simulink model "SWC_HALIN_type"  (R2021b)
settings: Solver=FixedStepDiscrete  StartTime=0.0  StopTime=10.0  FixedStep=0.005  RelTol=1e-3
values from neighbouring files (symbols this model uses):
  FALSE = boolean( 0 )    [vcu_local_hdr.m]    (also in vcu_local_hdrTA2.m)
  TRUE = boolean( 1 )    [vcu_local_hdr.m]    (also in vcu_local_hdrTA2.m)
undefined symbols (not defined in the file or in its folder): R_WDGCDD_CSOP_Call_Watchdog, R_WDGCDD_CSOP_Call_WDG_AppStart
libraries: halin x1, simulink x1
settings Model: DataDictionary=APPTypes.sldd  Creator=FVT23010  LastModifiedBy=FVT22063
settings DataIOCC: SaveFormat=StructureWithTime
settings OptimizationCC: DefaultParameterBehavior=Inlined  EnhancedBackFolding=on  PassReuseOutputArgsAs=Individual arguments  ZeroExternalMemoryAtStartup=off  ZeroInternalMemoryAtStartup=off  OptimizeBlockOrder=speed  DifferentSizesBufferReuse=on  OptimizationCustomize=off  EfficientTunableParamExpr=on
settings DebuggingCC: ParameterTunabilityLossMsg=error
settings HardwareCC: ProdBitPerPointer=32  ProdBitPerSizeT=32  ProdBitPerPtrDiffT=32  ProdLargestAtomicInteger=Long  ProdLargestAtomicFloat=Double  ProdWordSize=32  ProdLongLongMode=on  ProdHWDeviceType=ARM Compatible->ARM Cortex-M
settings ModelReferenceCC: ModelReferenceNumInstancesAllowed=Single
settings SFSimCC: MATLABDynamicMemAlloc=off
settings RTWCC: Description=AUTOSAR  SystemTargetFile=autosar.tlc  GenCodeOnly=on  TemplateMakefile=ert_default_tmf  PortableWordSizes=on
settings CodeAppCC: ForceParamTrailComments=on  IgnoreCustomStorageClasses=off  OperatorAnnotations=on  SimulinkDataObjDesc=on  SFDataObjDesc=on  InsertBlockDesc=on
settings STFCustomTargetCC: TargetLangStandard=C99 (ISO)  MultiwordLength=256  ParMdlRefBuildCompliant=on  CompOptLevelCompliant=on  IncludeMdlTerminateFcn=off  CombineOutputUpdateFcns=on  SuppressErrorStatus=on  ERTCustomFileBanners=on  SupportNonFinite=off  SupportComplex=off  SupportContinuousTime=off  SupportNonInlinedSFcns=off  RemoveResetFunc=on  MATLABClassNameForMDSCustomization=Simulink.SoftwareTarget.ERTCustomization  AutosarCompliant=on  GRTInterface=off  UseToolchainInfoCompliant=on  LookupTableObjectStructAxisOrder=2,1,3,4,...  LUTObjectStructOrderEvenSpacing=Size,Table,Breakpoints  SystemTargetFile=autosar.tlc
settings ERTTargetCC: TargetLangStandard=C99 (ISO)  ConcurrentExecutionCompliant=off  IncludeMdlTerminateFcn=off  SuppressErrorStatus=on  SupportNonFinite=off  SupportComplex=off  ModelStepFunctionPrototypeControlCompliant=off  CPPClassGenCompliant=off  AutosarCompliant=on  LookupTableObjectStructAxisOrder=2,1,3,4,...  LUTObjectStructOrderEvenSpacing=Size,Table,Breakpoints  GenerateASAP2=on  InlinedParameterPlacement=NonHierarchical  ERTCustomFileTemplate=example_file_process.tlc  ConvertIfToSwitch=off  SuppressUnreachableDefaultCases=off  BooleanTrueId=true_MatlabRTW  BooleanFalseId=false_MatlabRTW

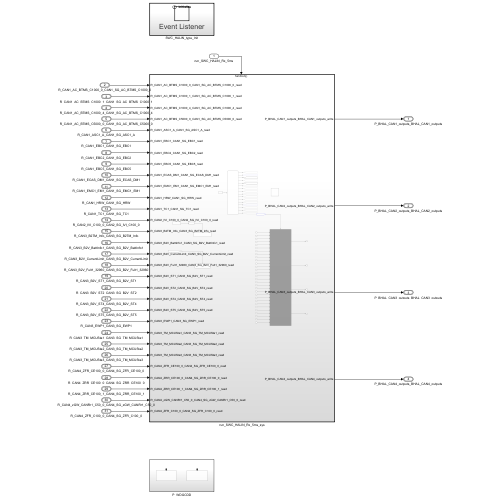
[thumbnail: Simulink's stored preview of the top-level diagram]
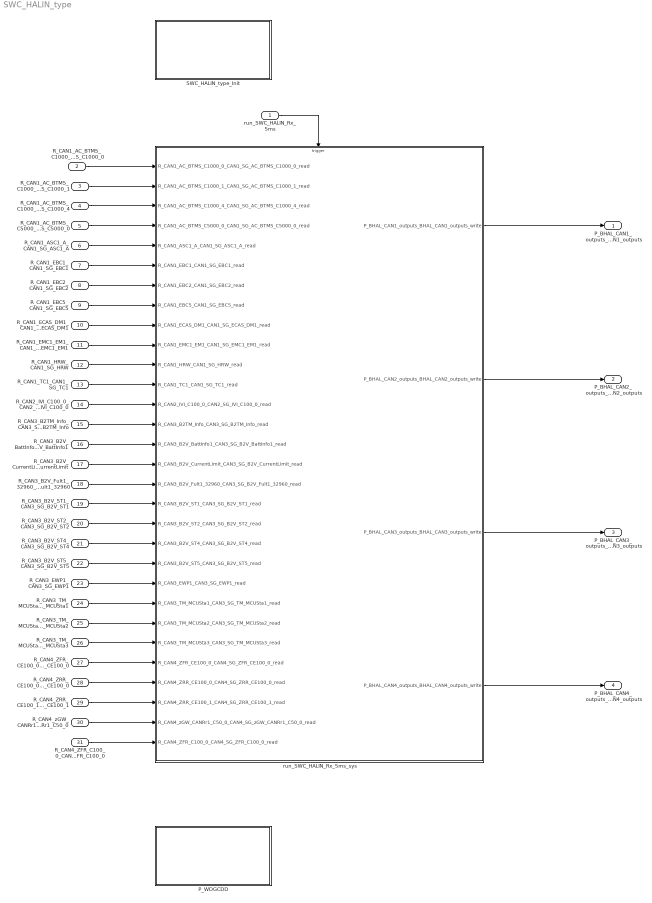
== system SWC_HALIN_type ==
  run_SWC_HALIN_Rx_5ms : Inport  SampleTime=0.005  OutputFunctionCall=on
  R_CAN1_AC_BTMS_C1000_0_CAN1_SG_AC_BTMS_C1000_0 : Inport  Port=2  OutDataTypeStr=Bus: DT_CAN1_SG_AC_BTMS_C1000_0  PortDimensions=1  BusOutputAsStruct=on
  R_CAN1_AC_BTMS_C1000_1_CAN1_SG_AC_BTMS_C1000_1 : Inport  Port=3  OutDataTypeStr=Bus: DT_CAN1_SG_AC_BTMS_C1000_1  PortDimensions=1  BusOutputAsStruct=on
  R_CAN1_AC_BTMS_C1000_4_CAN1_SG_AC_BTMS_C1000_4 : Inport  Port=4  OutDataTypeStr=Bus: DT_CAN1_SG_AC_BTMS_C1000_4  PortDimensions=1  BusOutputAsStruct=on
  R_CAN1_AC_BTMS_C5000_0_CAN1_SG_AC_BTMS_C5000_0 : Inport  Port=5  OutDataTypeStr=Bus: DT_CAN1_SG_AC_BTMS_C5000_0  PortDimensions=1  BusOutputAsStruct=on
  R_CAN1_ASC1_A_CAN1_SG_ASC1_A : Inport  Port=6  OutDataTypeStr=Bus: DT_CAN1_SG_ASC1_A  PortDimensions=1  BusOutputAsStruct=on
  R_CAN1_EBC1_CAN1_SG_EBC1 : Inport  Port=7  OutDataTypeStr=Bus: DT_CAN1_SG_EBC1  PortDimensions=1  BusOutputAsStruct=on
  R_CAN1_EBC2_CAN1_SG_EBC2 : Inport  Port=8  OutDataTypeStr=Bus: DT_CAN1_SG_EBC2  PortDimensions=1  BusOutputAsStruct=on
  R_CAN1_EBC5_CAN1_SG_EBC5 : Inport  Port=9  OutDataTypeStr=Bus: DT_CAN1_SG_EBC5  PortDimensions=1  BusOutputAsStruct=on
  R_CAN1_ECAS_DM1_CAN1_SG_ECAS_DM1 : Inport  Port=10  OutDataTypeStr=Bus: DT_CAN1_SG_ECAS_DM1  PortDimensions=1  BusOutputAsStruct=on
  R_CAN1_EMC1_EM1_CAN1_SG_EMC1_EM1 : Inport  Port=11  OutDataTypeStr=Bus: DT_CAN1_SG_EMC1_EM1  PortDimensions=1  BusOutputAsStruct=on
  R_CAN1_HRW_CAN1_SG_HRW : Inport  Port=12  OutDataTypeStr=Bus: DT_CAN1_SG_HRW  PortDimensions=1  BusOutputAsStruct=on
  R_CAN1_TC1_CAN1_SG_TC1 : Inport  Port=13  OutDataTypeStr=Bus: DT_CAN1_SG_TC1  PortDimensions=1  BusOutputAsStruct=on
  R_CAN2_IVI_C100_0_CAN2_SG_IVI_C100_0 : Inport  Port=14  OutDataTypeStr=Bus: DT_CAN2_SG_IVI_C100_0  PortDimensions=1  BusOutputAsStruct=on
  R_CAN3_B2TM_Info_CAN3_SG_B2TM_Info : Inport  Port=15  OutDataTypeStr=Bus: DT_CAN3_SG_B2TM_Info  PortDimensions=1  BusOutputAsStruct=on
  R_CAN3_B2V_BattInfo1_CAN3_SG_B2V_BattInfo1 : Inport  Port=16  OutDataTypeStr=Bus: DT_CAN3_SG_B2V_BattInfo1  PortDimensions=1  BusOutputAsStruct=on
  R_CAN3_B2V_CurrentLimit_CAN3_SG_B2V_CurrentLimit : Inport  Port=17  OutDataTypeStr=Bus: DT_CAN3_SG_B2V_CurrentLimit  PortDimensions=1  BusOutputAsStruct=on
  R_CAN3_B2V_Fult1_32960_CAN3_SG_B2V_Fult1_32960 : Inport  Port=18  OutDataTypeStr=Bus: DT_CAN3_SG_B2V_Fult1_32960  PortDimensions=1  BusOutputAsStruct=on
  R_CAN3_B2V_ST1_CAN3_SG_B2V_ST1 : Inport  Port=19  OutDataTypeStr=Bus: DT_CAN3_SG_B2V_ST1  PortDimensions=1  BusOutputAsStruct=on
  R_CAN3_B2V_ST2_CAN3_SG_B2V_ST2 : Inport  Port=20  OutDataTypeStr=Bus: DT_CAN3_SG_B2V_ST2  PortDimensions=1  BusOutputAsStruct=on
  R_CAN3_B2V_ST4_CAN3_SG_B2V_ST4 : Inport  Port=21  OutDataTypeStr=Bus: DT_CAN3_SG_B2V_ST4  PortDimensions=1  BusOutputAsStruct=on
  R_CAN3_B2V_ST5_CAN3_SG_B2V_ST5 : Inport  Port=22  OutDataTypeStr=Bus: DT_CAN3_SG_B2V_ST5  PortDimensions=1  BusOutputAsStruct=on
  R_CAN3_EWP1_CAN3_SG_EWP1 : Inport  Port=23  OutDataTypeStr=Bus: DT_CAN3_SG_EWP1  PortDimensions=1  BusOutputAsStruct=on
  R_CAN3_TM_MCUSta1_CAN3_SG_TM_MCUSta1 : Inport  Port=24  OutDataTypeStr=Bus: DT_CAN3_SG_TM_MCUSta1  PortDimensions=1  BusOutputAsStruct=on
  R_CAN3_TM_MCUSta2_CAN3_SG_TM_MCUSta2 : Inport  Port=25  OutDataTypeStr=Bus: DT_CAN3_SG_TM_MCUSta2  PortDimensions=1  BusOutputAsStruct=on
  R_CAN3_TM_MCUSta3_CAN3_SG_TM_MCUSta3 : Inport  Port=26  OutDataTypeStr=Bus: DT_CAN3_SG_TM_MCUSta3  PortDimensions=1  BusOutputAsStruct=on
  R_CAN4_ZFR_CE100_0_CAN4_SG_ZFR_CE100_0 : Inport  Port=27  OutDataTypeStr=Bus: DT_CAN4_SG_ZFR_CE100_0  PortDimensions=1  BusOutputAsStruct=on
  R_CAN4_ZRR_CE100_0_CAN4_SG_ZRR_CE100_0 : Inport  Port=28  OutDataTypeStr=Bus: DT_CAN4_SG_ZRR_CE100_0  PortDimensions=1  BusOutputAsStruct=on
  R_CAN4_ZRR_CE100_1_CAN4_SG_ZRR_CE100_1 : Inport  Port=29  OutDataTypeStr=Bus: DT_CAN4_SG_ZRR_CE100_1  PortDimensions=1  BusOutputAsStruct=on
  R_CAN4_zGW_CANRr1_C50_0_CAN4_SG_zGW_CANRr1_C50_0 : Inport  Port=30  OutDataTypeStr=Bus: DT_CAN4_SG_zGW_CANRr1_C50_0  PortDimensions=1  BusOutputAsStruct=on
  R_CAN4_ZFR_C100_0_CAN4_SG_ZFR_C100_0 : Inport  Port=31  OutDataTypeStr=Bus: DT_CAN4_SG_ZFR_C100_0  PortDimensions=1  BusOutputAsStruct=on
  P_WDGCDD : Subsystem
  SWC_HALIN_type_Init : Subsystem
  run_SWC_HALIN_Rx_5ms_sys : Subsystem
  P_BHAL_CAN1_outputs_BHAL_CAN1_outputs : Outport  OutDataTypeStr=Bus: BHAL_CAN1_outputs  PortDimensions=1  BusOutputAsStruct=on
  P_BHAL_CAN2_outputs_BHAL_CAN2_outputs : Outport  Port=2  OutDataTypeStr=Bus: BHAL_CAN2_outputs  PortDimensions=1  BusOutputAsStruct=on
  P_BHAL_CAN3_outputs_BHAL_CAN3_outputs : Outport  Port=3  OutDataTypeStr=Bus: BHAL_CAN3_outputs  PortDimensions=1  BusOutputAsStruct=on
  P_BHAL_CAN4_outputs_BHAL_CAN4_outputs : Outport  Port=4  OutDataTypeStr=Bus: BHAL_CAN4_outputs  PortDimensions=1  BusOutputAsStruct=on
  wires:
  R_CAN1_AC_BTMS_C1000_0_CAN1_SG_AC_BTMS_C1000_0/1 -> run_SWC_HALIN_Rx_5ms_sys/1(R_CAN1_AC_BTMS_C1000_0_CAN1_SG_AC_BTMS_C1000_0_read)
  R_CAN1_AC_BTMS_C1000_1_CAN1_SG_AC_BTMS_C1000_1/1 -> run_SWC_HALIN_Rx_5ms_sys/2(R_CAN1_AC_BTMS_C1000_1_CAN1_SG_AC_BTMS_C1000_1_read)
  R_CAN1_AC_BTMS_C1000_4_CAN1_SG_AC_BTMS_C1000_4/1 -> run_SWC_HALIN_Rx_5ms_sys/3(R_CAN1_AC_BTMS_C1000_4_CAN1_SG_AC_BTMS_C1000_4_read)
  R_CAN1_AC_BTMS_C5000_0_CAN1_SG_AC_BTMS_C5000_0/1 -> run_SWC_HALIN_Rx_5ms_sys/4(R_CAN1_AC_BTMS_C5000_0_CAN1_SG_AC_BTMS_C5000_0_read)
  R_CAN1_ASC1_A_CAN1_SG_ASC1_A/1 -> run_SWC_HALIN_Rx_5ms_sys/5(R_CAN1_ASC1_A_CAN1_SG_ASC1_A_read)
  R_CAN1_EBC1_CAN1_SG_EBC1/1 -> run_SWC_HALIN_Rx_5ms_sys/6(R_CAN1_EBC1_CAN1_SG_EBC1_read)
  R_CAN1_EBC2_CAN1_SG_EBC2/1 -> run_SWC_HALIN_Rx_5ms_sys/7(R_CAN1_EBC2_CAN1_SG_EBC2_read)
  R_CAN1_EBC5_CAN1_SG_EBC5/1 -> run_SWC_HALIN_Rx_5ms_sys/8(R_CAN1_EBC5_CAN1_SG_EBC5_read)
  R_CAN1_ECAS_DM1_CAN1_SG_ECAS_DM1/1 -> run_SWC_HALIN_Rx_5ms_sys/9(R_CAN1_ECAS_DM1_CAN1_SG_ECAS_DM1_read)
  R_CAN1_EMC1_EM1_CAN1_SG_EMC1_EM1/1 -> run_SWC_HALIN_Rx_5ms_sys/10(R_CAN1_EMC1_EM1_CAN1_SG_EMC1_EM1_read)
  R_CAN1_HRW_CAN1_SG_HRW/1 -> run_SWC_HALIN_Rx_5ms_sys/11(R_CAN1_HRW_CAN1_SG_HRW_read)
  R_CAN1_TC1_CAN1_SG_TC1/1 -> run_SWC_HALIN_Rx_5ms_sys/12(R_CAN1_TC1_CAN1_SG_TC1_read)
  R_CAN2_IVI_C100_0_CAN2_SG_IVI_C100_0/1 -> run_SWC_HALIN_Rx_5ms_sys/13(R_CAN2_IVI_C100_0_CAN2_SG_IVI_C100_0_read)
  R_CAN3_B2TM_Info_CAN3_SG_B2TM_Info/1 -> run_SWC_HALIN_Rx_5ms_sys/14(R_CAN3_B2TM_Info_CAN3_SG_B2TM_Info_read)
  R_CAN3_B2V_BattInfo1_CAN3_SG_B2V_BattInfo1/1 -> run_SWC_HALIN_Rx_5ms_sys/15(R_CAN3_B2V_BattInfo1_CAN3_SG_B2V_BattInfo1_read)
  R_CAN3_B2V_CurrentLimit_CAN3_SG_B2V_CurrentLimit/1 -> run_SWC_HALIN_Rx_5ms_sys/16(R_CAN3_B2V_CurrentLimit_CAN3_SG_B2V_CurrentLimit_read)
  R_CAN3_B2V_Fult1_32960_CAN3_SG_B2V_Fult1_32960/1 -> run_SWC_HALIN_Rx_5ms_sys/17(R_CAN3_B2V_Fult1_32960_CAN3_SG_B2V_Fult1_32960_read)
  R_CAN3_B2V_ST1_CAN3_SG_B2V_ST1/1 -> run_SWC_HALIN_Rx_5ms_sys/18(R_CAN3_B2V_ST1_CAN3_SG_B2V_ST1_read)
  R_CAN3_B2V_ST2_CAN3_SG_B2V_ST2/1 -> run_SWC_HALIN_Rx_5ms_sys/19(R_CAN3_B2V_ST2_CAN3_SG_B2V_ST2_read)
  R_CAN3_B2V_ST4_CAN3_SG_B2V_ST4/1 -> run_SWC_HALIN_Rx_5ms_sys/20(R_CAN3_B2V_ST4_CAN3_SG_B2V_ST4_read)
  R_CAN3_B2V_ST5_CAN3_SG_B2V_ST5/1 -> run_SWC_HALIN_Rx_5ms_sys/21(R_CAN3_B2V_ST5_CAN3_SG_B2V_ST5_read)
  R_CAN3_EWP1_CAN3_SG_EWP1/1 -> run_SWC_HALIN_Rx_5ms_sys/22(R_CAN3_EWP1_CAN3_SG_EWP1_read)
  R_CAN3_TM_MCUSta1_CAN3_SG_TM_MCUSta1/1 -> run_SWC_HALIN_Rx_5ms_sys/23(R_CAN3_TM_MCUSta1_CAN3_SG_TM_MCUSta1_read)
  R_CAN3_TM_MCUSta2_CAN3_SG_TM_MCUSta2/1 -> run_SWC_HALIN_Rx_5ms_sys/24(R_CAN3_TM_MCUSta2_CAN3_SG_TM_MCUSta2_read)
  R_CAN3_TM_MCUSta3_CAN3_SG_TM_MCUSta3/1 -> run_SWC_HALIN_Rx_5ms_sys/25(R_CAN3_TM_MCUSta3_CAN3_SG_TM_MCUSta3_read)
  R_CAN4_ZFR_CE100_0_CAN4_SG_ZFR_CE100_0/1 -> run_SWC_HALIN_Rx_5ms_sys/26(R_CAN4_ZFR_CE100_0_CAN4_SG_ZFR_CE100_0_read)
  R_CAN4_ZRR_CE100_0_CAN4_SG_ZRR_CE100_0/1 -> run_SWC_HALIN_Rx_5ms_sys/27(R_CAN4_ZRR_CE100_0_CAN4_SG_ZRR_CE100_0_read)
  R_CAN4_ZRR_CE100_1_CAN4_SG_ZRR_CE100_1/1 -> run_SWC_HALIN_Rx_5ms_sys/28(R_CAN4_ZRR_CE100_1_CAN4_SG_ZRR_CE100_1_read)
  R_CAN4_zGW_CANRr1_C50_0_CAN4_SG_zGW_CANRr1_C50_0/1 -> run_SWC_HALIN_Rx_5ms_sys/29(R_CAN4_zGW_CANRr1_C50_0_CAN4_SG_zGW_CANRr1_C50_0_read)
  run_SWC_HALIN_Rx_5ms_sys/1(P_BHAL_CAN1_outputs_BHAL_CAN1_outputs_write) -> P_BHAL_CAN1_outputs_BHAL_CAN1_outputs/1
  run_SWC_HALIN_Rx_5ms_sys/2(P_BHAL_CAN2_outputs_BHAL_CAN2_outputs_write) -> P_BHAL_CAN2_outputs_BHAL_CAN2_outputs/1
  run_SWC_HALIN_Rx_5ms_sys/3(P_BHAL_CAN3_outputs_BHAL_CAN3_outputs_write) -> P_BHAL_CAN3_outputs_BHAL_CAN3_outputs/1
  run_SWC_HALIN_Rx_5ms_sys/4(P_BHAL_CAN4_outputs_BHAL_CAN4_outputs_write) -> P_BHAL_CAN4_outputs_BHAL_CAN4_outputs/1
  run_SWC_HALIN_Rx_5ms/1 -> run_SWC_HALIN_Rx_5ms_sys/Trigger
  R_CAN4_ZFR_C100_0_CAN4_SG_ZFR_C100_0/1 -> run_SWC_HALIN_Rx_5ms_sys/30(R_CAN4_ZFR_C100_0_CAN4_SG_ZFR_C100_0_read)

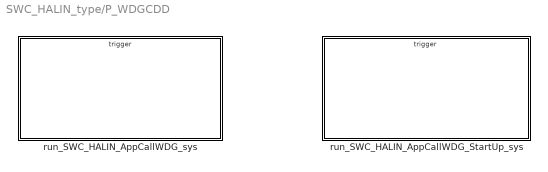
== system SWC_HALIN_type/P_WDGCDD ==
  run_SWC_HALIN_AppCallWDG_StartUp_sys : Subsystem
  run_SWC_HALIN_AppCallWDG_sys : Subsystem

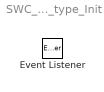
== system SWC_HALIN_type/SWC_HALIN_type_Init ==
  Event Listener : EventListener  EventName=reset

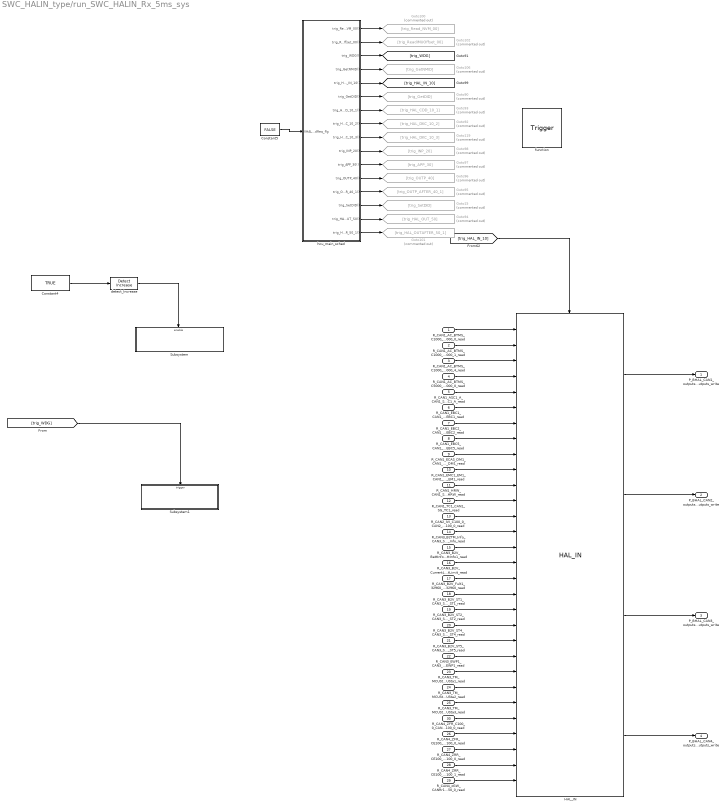
== system SWC_HALIN_type/run_SWC_HALIN_Rx_5ms_sys ==
  R_CAN1_AC_BTMS_C1000_0_CAN1_SG_AC_BTMS_C1000_0_read : Inport
  R_CAN1_AC_BTMS_C1000_1_CAN1_SG_AC_BTMS_C1000_1_read : Inport  Port=2
  R_CAN1_AC_BTMS_C1000_4_CAN1_SG_AC_BTMS_C1000_4_read : Inport  Port=3
  R_CAN1_AC_BTMS_C5000_0_CAN1_SG_AC_BTMS_C5000_0_read : Inport  Port=4
  R_CAN1_ASC1_A_CAN1_SG_ASC1_A_read : Inport  Port=5
  R_CAN1_EBC1_CAN1_SG_EBC1_read : Inport  Port=6
  R_CAN1_EBC2_CAN1_SG_EBC2_read : Inport  Port=7
  R_CAN1_EBC5_CAN1_SG_EBC5_read : Inport  Port=8
  R_CAN1_ECAS_DM1_CAN1_SG_ECAS_DM1_read : Inport  Port=9
  R_CAN1_EMC1_EM1_CAN1_SG_EMC1_EM1_read : Inport  Port=10
  R_CAN1_HRW_CAN1_SG_HRW_read : Inport  Port=11
  R_CAN1_TC1_CAN1_SG_TC1_read : Inport  Port=12
  R_CAN2_IVI_C100_0_CAN2_SG_IVI_C100_0_read : Inport  Port=13
  R_CAN3_B2TM_Info_CAN3_SG_B2TM_Info_read : Inport  Port=14
  R_CAN3_B2V_BattInfo1_CAN3_SG_B2V_BattInfo1_read : Inport  Port=15
  R_CAN3_B2V_CurrentLimit_CAN3_SG_B2V_CurrentLimit_read : Inport  Port=16
  R_CAN3_B2V_Fult1_32960_CAN3_SG_B2V_Fult1_32960_read : Inport  Port=17
  R_CAN3_B2V_ST1_CAN3_SG_B2V_ST1_read : Inport  Port=18
  R_CAN3_B2V_ST2_CAN3_SG_B2V_ST2_read : Inport  Port=19
  R_CAN3_B2V_ST4_CAN3_SG_B2V_ST4_read : Inport  Port=20
  R_CAN3_B2V_ST5_CAN3_SG_B2V_ST5_read : Inport  Port=21
  R_CAN3_EWP1_CAN3_SG_EWP1_read : Inport  Port=22
  R_CAN3_TM_MCUSta1_CAN3_SG_TM_MCUSta1_read : Inport  Port=23
  R_CAN3_TM_MCUSta2_CAN3_SG_TM_MCUSta2_read : Inport  Port=24
  R_CAN3_TM_MCUSta3_CAN3_SG_TM_MCUSta3_read : Inport  Port=25
  R_CAN4_ZFR_CE100_0_CAN4_SG_ZFR_CE100_0_read : Inport  Port=26
  R_CAN4_ZRR_CE100_0_CAN4_SG_ZRR_CE100_0_read : Inport  Port=27
  R_CAN4_ZRR_CE100_1_CAN4_SG_ZRR_CE100_1_read : Inport  Port=28
  R_CAN4_zGW_CANRr1_C50_0_CAN4_SG_zGW_CANRr1_C50_0_read : Inport  Port=29
  R_CAN4_ZFR_C100_0_CAN4_SG_ZFR_C100_0_read : Inport  Port=30
  function : TriggerPort  TriggerType=function-call  VariantControl=(inherit)  SampleTimeType=periodic  SampleTime=-1
  Constant4 : Constant  Value=TRUE
  Constant5 : Constant  Value=FALSE
  Goto100 : Goto  Commented=on  GotoTag=trig_Read_NVM_00
  Goto101 : Goto  Commented=on  GotoTag=trig_HAL_OUTAFTER_50_1
  Goto102 : Goto  Commented=on  GotoTag=trig_ReadIMUOffset_00
  Goto106 : Goto  Commented=on  GotoTag=trig_GetNMID
  Goto119 : Goto  Commented=on  GotoTag=trig_HAL_DKC_10_3
  Goto15 : Goto  Commented=on  GotoTag=trig_SetDID
  Goto90 : Goto  Commented=on  GotoTag=trig_GetDID
  Goto92 : Goto  Commented=on  GotoTag=trig_HAL_DKC_10_2
  Goto93 : Goto  Commented=on  GotoTag=trig_HAL_CDD_10_1
  Goto94 : Goto  Commented=on  GotoTag=trig_HAL_OUT_50
  Goto95 : Goto  Commented=on  GotoTag=trig_OUTP_AFTER_40_1
  Goto96 : Goto  Commented=on  GotoTag=trig_OUTP_40
  Goto97 : Goto  Commented=on  GotoTag=trig_APP_30
  Goto98 : Goto  Commented=on  GotoTag=trig_INP_20
  HAL_IN : halin/HAL_IN  SystemSampleTime=-1  VariantActivationTime=update diagram  Latency=0  AutoFrameSizeCalculation=off
  Subsystem : Subsystem
  Subsystem1 : Subsystem
  detect_Increase : simulink/Logic and Bit Operations/Detect Increase  vinit=0.0  OutDataTypeStr=boolean
  hcu_main_sched : Stateflow chart  TreatAsAtomicUnit=on
  P_BHAL_CAN1_outputs_BHAL_CAN1_outputs_write : Outport
  P_BHAL_CAN2_outputs_BHAL_CAN2_outputs_write : Outport  Port=2
  P_BHAL_CAN3_outputs_BHAL_CAN3_outputs_write : Outport  Port=3
  P_BHAL_CAN4_outputs_BHAL_CAN4_outputs_write : Outport  Port=4
  wires:
  detect_Increase/1 -> Subsystem/Enable
  Constant4/1 -> detect_Increase/1
  [trig_WDG] -> Subsystem1/Trigger
  hcu_main_sched/4(trig_GetNMID()) -> Goto106/1
  hcu_main_sched/12(trig_OUTP_40()) -> Goto96/1
  hcu_main_sched/3(trig_WDG()) -> [trig_WDG]
  hcu_main_sched/8(trig_HAL_DKC_10_2()) -> Goto92/1
  hcu_main_sched/15(trig_HAL_OUT_50()) -> Goto94/1
  hcu_main_sched/6(trig_GetDID()) -> Goto90/1
  hcu_main_sched/1(trig_Read_NVM_00()) -> Goto100/1
  hcu_main_sched/5(trig_HAL_IN_10()) -> [trig_HAL_IN_10]
  Constant5/1 -> hcu_main_sched/1(VHAL_FusionSchedReq_flg)
  hcu_main_sched/13(trig_OUTP_AFTER_40_1()) -> Goto95/1
  hcu_main_sched/7(trig_HAL_CDD_10_1()) -> Goto93/1
  hcu_main_sched/14(trig_SetDID()) -> Goto15/1
  hcu_main_sched/10(trig_INP_20()) -> Goto98/1
  hcu_main_sched/11(trig_APP_30()) -> Goto97/1
  hcu_main_sched/2(trig_ReadIMUOffset_00()) -> Goto102/1
  hcu_main_sched/9(trig_HAL_DKC_10_3()) -> Goto119/1
  hcu_main_sched/16(trig_HAL_OUTAFTER_50_1()) -> Goto101/1
  [trig_HAL_IN_10] -> HAL_IN/Trigger
  R_CAN1_ECAS_DM1_CAN1_SG_ECAS_DM1_read/1 -> HAL_IN/9
  R_CAN1_EMC1_EM1_CAN1_SG_EMC1_EM1_read/1 -> HAL_IN/10
  R_CAN1_EBC1_CAN1_SG_EBC1_read/1 -> HAL_IN/6
  R_CAN1_EBC2_CAN1_SG_EBC2_read/1 -> HAL_IN/7
  R_CAN1_EBC5_CAN1_SG_EBC5_read/1 -> HAL_IN/8
  R_CAN1_HRW_CAN1_SG_HRW_read/1 -> HAL_IN/11
  R_CAN1_TC1_CAN1_SG_TC1_read/1 -> HAL_IN/12
  R_CAN2_IVI_C100_0_CAN2_SG_IVI_C100_0_read/1 -> HAL_IN/13
  R_CAN1_AC_BTMS_C5000_0_CAN1_SG_AC_BTMS_C5000_0_read/1 -> HAL_IN/4
  R_CAN1_ASC1_A_CAN1_SG_ASC1_A_read/1 -> HAL_IN/5
  R_CAN3_B2TM_Info_CAN3_SG_B2TM_Info_read/1 -> HAL_IN/14
  R_CAN3_B2V_BattInfo1_CAN3_SG_B2V_BattInfo1_read/1 -> HAL_IN/15
  R_CAN1_AC_BTMS_C1000_0_CAN1_SG_AC_BTMS_C1000_0_read/1 -> HAL_IN/1
  R_CAN1_AC_BTMS_C1000_1_CAN1_SG_AC_BTMS_C1000_1_read/1 -> HAL_IN/2
  R_CAN1_AC_BTMS_C1000_4_CAN1_SG_AC_BTMS_C1000_4_read/1 -> HAL_IN/3
  R_CAN3_B2V_CurrentLimit_CAN3_SG_B2V_CurrentLimit_read/1 -> HAL_IN/16
  R_CAN3_B2V_Fult1_32960_CAN3_SG_B2V_Fult1_32960_read/1 -> HAL_IN/17
  R_CAN3_B2V_ST1_CAN3_SG_B2V_ST1_read/1 -> HAL_IN/18
  R_CAN3_B2V_ST2_CAN3_SG_B2V_ST2_read/1 -> HAL_IN/19
  R_CAN3_B2V_ST4_CAN3_SG_B2V_ST4_read/1 -> HAL_IN/20
  R_CAN3_B2V_ST5_CAN3_SG_B2V_ST5_read/1 -> HAL_IN/21
  R_CAN3_EWP1_CAN3_SG_EWP1_read/1 -> HAL_IN/22
  R_CAN3_TM_MCUSta1_CAN3_SG_TM_MCUSta1_read/1 -> HAL_IN/23
  R_CAN3_TM_MCUSta2_CAN3_SG_TM_MCUSta2_read/1 -> HAL_IN/24
  R_CAN3_TM_MCUSta3_CAN3_SG_TM_MCUSta3_read/1 -> HAL_IN/25
  R_CAN4_ZFR_CE100_0_CAN4_SG_ZFR_CE100_0_read/1 -> HAL_IN/27
  R_CAN4_ZRR_CE100_0_CAN4_SG_ZRR_CE100_0_read/1 -> HAL_IN/28
  R_CAN4_ZRR_CE100_1_CAN4_SG_ZRR_CE100_1_read/1 -> HAL_IN/29
  R_CAN4_zGW_CANRr1_C50_0_CAN4_SG_zGW_CANRr1_C50_0_read/1 -> HAL_IN/30
  HAL_IN/1 -> P_BHAL_CAN1_outputs_BHAL_CAN1_outputs_write/1
  HAL_IN/2 -> P_BHAL_CAN2_outputs_BHAL_CAN2_outputs_write/1
  HAL_IN/3 -> P_BHAL_CAN3_outputs_BHAL_CAN3_outputs_write/1
  HAL_IN/4 -> P_BHAL_CAN4_outputs_BHAL_CAN4_outputs_write/1
  R_CAN4_ZFR_C100_0_CAN4_SG_ZFR_C100_0_read/1 -> HAL_IN/26

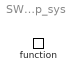
== system SWC_HALIN_type/P_WDGCDD/run_SWC_HALIN_AppCallWDG_StartUp_sys ==
  function : TriggerPort  TriggerType=function-call  IsSimulinkFunction=on  FunctionName=run_SWC_HALIN_AppCallWDG_StartUp  VariantControl=(inherit)

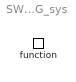
== system SWC_HALIN_type/P_WDGCDD/run_SWC_HALIN_AppCallWDG_sys ==
  function : TriggerPort  TriggerType=function-call  IsSimulinkFunction=on  FunctionName=run_SWC_HALIN_AppCallWDG  VariantControl=(inherit)

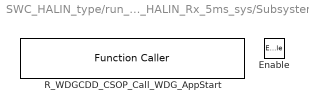
== system SWC_HALIN_type/run_SWC_HALIN_Rx_5ms_sys/Subsystem ==
  Enable : EnablePort
  R_WDGCDD_CSOP_Call_WDG_AppStart : FunctionCaller  FunctionPrototype=R_WDGCDD_CSOP_Call_WDG_AppStart()

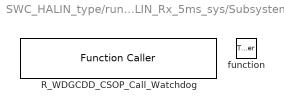
== system SWC_HALIN_type/run_SWC_HALIN_Rx_5ms_sys/Subsystem1 ==
  function : TriggerPort  TriggerType=function-call  VariantControl=(inherit)
  R_WDGCDD_CSOP_Call_Watchdog : FunctionCaller  FunctionPrototype=R_WDGCDD_CSOP_Call_Watchdog()

== stateflow chart SWC_HALIN_type/run_SWC_HALIN_Rx_5ms_sys/hcu_main_sched ==
  state Main_Scheduler
    (default) -> (junction 31) : {
        |   Sys_Init_done = FALSE;
        |   trig_Read_NVM_00;
        |   trig_ReadIMUOffset_00;
        | }
    Main_Scheduler -> (junction 31) : {Sys_Init_done = TRUE;}
    (junction 31) -> (junction 34) [order 1] : [
        |    Sys_Init_done &&...
        |    !VHAL_FusionSchedReq_flg
        | ]
    (junction 31) -> (junction 38) [order 2]
    (junction 34) -> (junction 36) : {
        |     trig_WDG;
        |     trig_GetNMID;
        |     trig_HAL_IN_10;
        |     trig_GetDID;
        |     trig_HAL_CDD_10_1;
        |     trig_HAL_DKC_10_2;
        |     trig_HAL_DKC_10_3;
        |     trig_INP_20;
        |     trig_APP_30;
        |     trig_OUTP_40;
        |     trig_OUTP_AFTER_40_1;
        |     trig_SetDID;
        |     trig_HAL_OUT_50;
        |     trig_HAL_OUTAFTER_50_1;
        |    }
    (junction 36) -> (junction 38)
  (default) -> Main_Scheduler
  data: VHAL_FusionSchedReq_flg input; Sys_Init_done local double; FALSE parameter; TRUE parameter
  events: trig_Read_NVM_00 output FUNCTION_CALL_EVENT; trig_ReadIMUOffset_00 output FUNCTION_CALL_EVENT; trig_WDG output FUNCTION_CALL_EVENT; trig_GetNMID output FUNCTION_CALL_EVENT; trig_HAL_IN_10 output FUNCTION_CALL_EVENT; trig_GetDID output FUNCTION_CALL_EVENT; trig_HAL_CDD_10_1 output FUNCTION_CALL_EVENT; trig_HAL_DKC_10_2 output FUNCTION_CALL_EVENT; trig_HAL_DKC_10_3 output FUNCTION_CALL_EVENT; trig_INP_20 output FUNCTION_CALL_EVENT; trig_APP_30 output FUNCTION_CALL_EVENT; trig_OUTP_40 output FUNCTION_CALL_EVENT; trig_OUTP_AFTER_40_1 output FUNCTION_CALL_EVENT; trig_SetDID output FUNCTION_CALL_EVENT; trig_HAL_OUT_50 output FUNCTION_CALL_EVENT; trig_HAL_OUTAFTER_50_1 output FUNCTION_CALL_EVENT
